simulink model "Distribuition"  (R2024a)
settings: Solver=VariableStepAuto  StartTime=0.0  StopTime=10.0  RelTol=1e-3
InitFcn:
  | % Exemplo no Windows, usando pscp (PuTTY scp) ou scp no Linux/macOS
  | chave = 'C:/Users/guilh/OneDrive/Área de Trabalho/matlab-Gemeo/Sombra_Distribution/Matlab_conect/id_rsa_matlab';
  | usuario = 'root';
  | ip = '200.145.26.206';
  | arquivo_remoto = '/root/ProjetoGemeo/AAS/Distribution/Variables.csv';
  | arquivo_local = 'Variables.csv';
  | 
  | % Comando scp para baixar arquivo usando chave privada
  | cmd = sprintf('scp -i "%s" %s@%s:"%s" "%s"', chave, usuario, ip, arquivo_remoto);
  | 
  | % Executar comando no sistema
  | [status, cmdout] = system(cmd);
  | 
  | if status == 0
  |     disp('Download concluído via SCP externo!');
  | else
  |     disp('Erro ao executar SCP:');
  |     disp(cmdout);
  | end
  | 
  | tabela = readtable('Variables.csv', 'Delimiter', ';');
  | nomesVariaveis = tabela.Variable;
libraries: opclib x1, opcualib x1
settings Model: Creator=guilh  LastModifiedBy=guilh

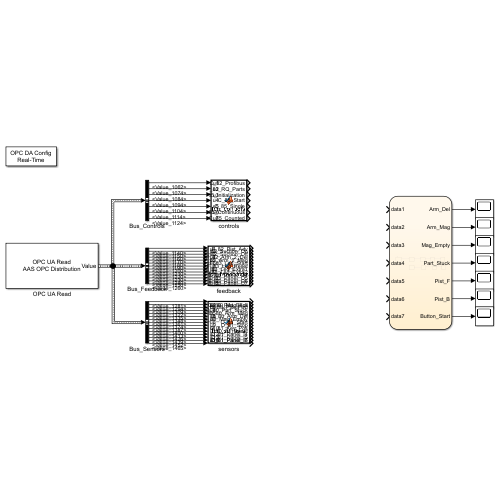
[thumbnail: Simulink's stored preview of the top-level diagram]
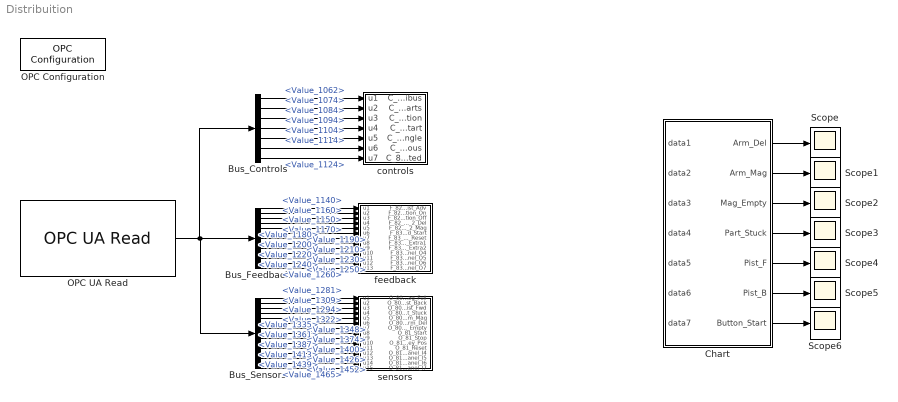
== system Distribuition ==
  Bus_Controls : BusSelector  OutputSignals=Value_1062,Value_1074,Value_1084,Value_1094,Value_1104,Value_1114,Value_1124
  Bus_Feedback : BusSelector  OutputSignals=Value_1140,Value_1150,Value_1160,Value_1170,Value_1180,Value_1190,Value_1200,Value_1210,Value_1220,Value_1230,Value_1240,Value_1250,Value_1260
  Bus_Sensors : BusSelector  OutputSignals=Value_1281,Value_1294,Value_1309,Value_1322,Value_1335,Value_1348,Value_1361,Value_1374,Value_1387,Value_1400,Value_1413,Value_1426,Value_1439,Value_1452,Value_1465
  Chart : Stateflow chart  TreatAsAtomicUnit=on
  OPC Configuration : opclib/OPC Configuration  errMissingItems=Error  errReadWrite=Warn  errShutdown=Error  errRTViolation=Warn  rtEnable=on  speedup=1  showLatency=off  beingUsed=on
  OPC UA Read : opcualib/OPC UA Read  SelectedServer=AAS OPC Distribution  ServerList=AAS OPC Distribution  NodeList={ '1', 'Value', '6', '1062', '1'; '2', 'Value', '6', '1074', '1'; '3', 'Value', '6', '1084', '1'; '4', 'Value', '6', '1094', '1'; '5', 'Value', '6', '1104', '1'; '6', 'Value', '6', '1114', '1'; '7', 'Value', '6', '1124', '1'; '8', 'Value', '6', '1140', '1'; '9', 'Value', '6', '1150', '1'; '10', 'Value', '6', '1160', '1'; '11', 'Value', '6', '1170', '1'; '12', 'Value', '6', '1180', '1'; '13', 'Value', '6', '1190', '1'; '14', 'Value', '6', '1200', '1'; '15', 'Value', '6', '1210', '1'; '16', 'Value', '6', '1220', '1'; '17', 'Value', '6', '1230', '1'; '18', 'Value', '6', '1240', '1'; '19', 'Value', '6', '1250', '1'; '20', 'Value', '6', '1260', '1'; '21', 'Value', '6', '1281', '1'; '22', 'Value', '6', '1294', '1'; '23', 'Value', '6', '1309', '1'; '24', 'Value', '6', '1322', '1'; '25', 'Value', '6', '1335', '1'; '26', 'Value', '6', '1348', '1'; '27', 'Value', '6', '1361', '1'; '28', 'Value', '6', '1374', '1'; '29', 'Value', '6', '1387', '1'; '30', 'Value', '6', '1400', '1'; '31', 'Value', '6', '1413', '1'; '32', 'Value', '6', '1426', '1'; '33', 'Value', '6', '1439', '1'; '34', 'Value', '6', '1452', '1'; '35', 'Value', '6', '1465', '1' }  ShowQualityPort=off  ShowTimestampPort=off  ShowTimestampPortAs=Seconds since start  SampleTime=-1
  Scope{,1..6} (7 alike) : Scope
  controls : MATLAB Function  TreatAsAtomicUnit=on
  feedback : MATLAB Function  TreatAsAtomicUnit=on
  sensors : MATLAB Function  TreatAsAtomicUnit=on
  wires:
  Chart/1(Arm_Del) -> Scope/1
  Chart/2(Arm_Mag) -> Scope1/1
  Chart/3(Mag_Empty) -> Scope2/1
  Chart/4(Part_Stuck) -> Scope3/1
  Chart/5(Pist_F) -> Scope4/1
  Chart/6(Pist_B) -> Scope5/1
  Chart/7(Button_Start) -> Scope6/1
  OPC UA Read/1 -> Bus_Sensors/1, Bus_Feedback/1, Bus_Controls/1
  Bus_Controls/7 -> controls/7(u7)  "<Value_1124>"
  Bus_Controls/6 -> controls/6(u6)  "<Value_1114>"
  Bus_Controls/5 -> controls/5(u5)  "<Value_1104>"
  Bus_Controls/4 -> controls/4(u4)  "<Value_1094>"
  Bus_Controls/3 -> controls/3(u3)  "<Value_1084>"
  Bus_Controls/2 -> controls/2(u2)  "<Value_1074>"
  Bus_Controls/1 -> controls/1(u1)  "<Value_1062>"
  Bus_Feedback/1 -> feedback/1(u1)  "<Value_1140>"
  Bus_Feedback/2 -> feedback/2(u2)  "<Value_1150>"
  Bus_Feedback/3 -> feedback/3(u3)  "<Value_1160>"
  Bus_Feedback/4 -> feedback/4(u4)  "<Value_1170>"
  Bus_Feedback/5 -> feedback/5(u5)  "<Value_1180>"
  Bus_Feedback/6 -> feedback/6(u6)  "<Value_1190>"
  Bus_Feedback/7 -> feedback/7(u7)  "<Value_1200>"
  Bus_Feedback/8 -> feedback/8(u8)  "<Value_1210>"
  Bus_Feedback/9 -> feedback/9(u9)  "<Value_1220>"
  Bus_Feedback/10 -> feedback/10(u10)  "<Value_1230>"
  Bus_Feedback/11 -> feedback/11(u11)  "<Value_1240>"
  Bus_Feedback/12 -> feedback/12(u12)  "<Value_1250>"
  Bus_Feedback/13 -> feedback/13(u13)  "<Value_1260>"
  Bus_Sensors/1 -> sensors/1(u1)  "<Value_1281>"
  Bus_Sensors/2 -> sensors/2(u2)  "<Value_1294>"
  Bus_Sensors/3 -> sensors/3(u3)  "<Value_1309>"
  Bus_Sensors/4 -> sensors/4(u4)  "<Value_1322>"
  Bus_Sensors/5 -> sensors/5(u5)  "<Value_1335>"
  Bus_Sensors/6 -> sensors/6(u6)  "<Value_1348>"
  Bus_Sensors/7 -> sensors/7(u7)  "<Value_1361>"
  Bus_Sensors/8 -> sensors/8(u8)  "<Value_1374>"
  Bus_Sensors/9 -> sensors/9(u9)  "<Value_1387>"
  Bus_Sensors/10 -> sensors/10(u10)  "<Value_1400>"
  Bus_Sensors/11 -> sensors/11(u11)  "<Value_1413>"
  Bus_Sensors/12 -> sensors/12(u12)  "<Value_1426>"
  Bus_Sensors/13 -> sensors/13(u13)  "<Value_1439>"
  Bus_Sensors/14 -> sensors/14(u14)  "<Value_1452>"
  Bus_Sensors/15 -> sensors/15(u15)  "<Value_1465>"

== matlab function Distribuition/sensors ==
  data: u1 input; u2 input; u3 input; u4 input; u5 input; u6 input; u7 input; u8 input; u9 input; u10 input; u11 input; u12 input; u13 input; u14 input; u15 input; O_80_Mag_Full output; O_80_Pist_Back output; O_80_Pist_Fwd output; O_80_Part_Stuck output; O_80_Arm_Mag output; O_80_Arm_Del output; O_80_Mag_Empty output; O_81_Start output; O_81_Stop output; O_81_Key_Pos output; O_81_Reset output; O_81_Panel_I4 output; O_81_Panel_I5 output; O_81_Panel_I6 output; O_81_Panel_I7 output
function [O_80_Mag_Full,O_80_Pist_Back,O_80_Pist_Fwd,O_80_Part_Stuck,...
    O_80_Arm_Mag,O_80_Arm_Del,O_80_Mag_Empty,O_81_Start,O_81_Stop,...
    O_81_Key_Pos,O_81_Reset,O_81_Panel_I4,O_81_Panel_I5,O_81_Panel_I6,...
    O_81_Panel_I7] = fcn_sensors(u1,u2,u3,u4,u5,u6,u7,u8,u9,...
    u10,u11,u12,u13,u14,u15)

O_80_Mag_Full = u1;
O_80_Pist_Back = u2;
O_80_Pist_Fwd = u3;
O_80_Part_Stuck = u4;
O_80_Arm_Mag = u5;
O_80_Arm_Del = u6;
O_80_Mag_Empty = u7;
O_81_Start = u8;
O_81_Stop = u9;
O_81_Key_Pos = u10;
O_81_Reset = u11;
O_81_Panel_I4 = u12;
O_81_Panel_I5 = u13;
O_81_Panel_I6 = u14;
O_81_Panel_I7 = u15;

== matlab function Distribuition/feedback ==
  data: u1 input; F_82_Pist_Adv output; u2 input; u3 input; u4 input; u5 input; u6 input; u7 input; u8 input; u9 input; u10 input; u11 input; u12 input; u13 input; F_82_Suction_On output; F_82_Suction_Off output; F_82_Arm_2_Del output; F_82_Arm_2_Mag output; F_83_Led_Start output; F_83_Led_Reset output; F_83_Led_Extra1 output; F_83_Led_Extra2 output; F_83_Panel_O4 output; F_83_Panel_O5 output; F_83_Panel_O6 output; F_83_Panel_O7 output
function [F_82_Pist_Adv,F_82_Suction_On,F_82_Suction_Off,F_82_Arm_2_Del, ...
    F_82_Arm_2_Mag,F_83_Led_Start,F_83_Led_Reset,F_83_Led_Extra1,...
    F_83_Led_Extra2,F_83_Panel_O4,F_83_Panel_O5,F_83_Panel_O6,...
    F_83_Panel_O7] = fcn_feedbacks(u1,u2,u3,u4,u5,u6,u7,u8,u9,...
    u10,u11,u12,u13)

F_82_Pist_Adv = u1;
F_82_Suction_On = u2;
F_82_Suction_Off = u3;
F_82_Arm_2_Del = u4;
F_82_Arm_2_Mag = u5;
F_83_Led_Start = u6;
F_83_Led_Reset = u7;
F_83_Led_Extra1 = u8;
F_83_Led_Extra2 = u9;
F_83_Panel_O4 = u10;
F_83_Panel_O5 = u11;
F_83_Panel_O6 = u12;
F_83_Panel_O7 = u13;

== matlab function Distribuition/controls ==
  data: u1 input; u2 input; u3 input; u4 input; u5 input; u6 input; u7 input; C_82_Profibus output; C_83_RQ_Parts output; C_85_Initialization output; C_85_Start output; C_85_Single output; C_85_Continuous output; C_85_Counted output
function [C_82_Profibus, C_83_RQ_Parts, ...
    C_85_Initialization, C_85_Start, ...
    C_85_Single, C_85_Continuous, ...
    C_85_Counted] = fcn_controls(u1,u2,u3,u4,u5,u6,u7)

C_82_Profibus = u1;
C_83_RQ_Parts = u2;
C_85_Initialization = u3;
C_85_Start = u4;
C_85_Single = u5; 
C_85_Continuous = u6;
C_85_Counted = u7;

== stateflow chart Distribuition/Chart ==
  state Init
    entry:
    Button_Start = data7;
    Pist_B = data1;
    Pist_F = data2;
    Part_Stuck = data3;
    Arm_Mag = data4;
    Arm_Del = data5;
    Mag_Empty = data6;
  state Arm_2_Del
    entry:
    Pist_B = 1;
    Pist_F = 0;
    Part_Stuck = 0;
    Arm_Mag = 0;
    Arm_Del = 1;
    Mag_Empty = 0;
  state Pist_Fowd
    entry:
    Pist_B = 0;
    Pist_F = 1;
    Part_Stuck = 0;
    Arm_Mag = 0;
    Arm_Del = 1;
    Mag_Empty = 0;
  state Pist_Back
    entry:
    Pist_B = 1;
    Pist_F = 0;
    Part_Stuck = 0;
    Arm_Mag = 0;
    Arm_Del = 1;
    Mag_Empty = 0;
  state Arm_2_Mag
    entry:
    Pist_B = 1;
    Pist_F = 0;
    Part_Stuck = 0;
    Arm_Mag = 1;
    Arm_Del = 0;
    Mag_Empty = 0;
  state Arm_2_Mag1
    entry:
    Button_Start = 0;
    Pist_B = 1;
    Pist_F = 0;
    Part_Stuck = 0;
    Arm_Mag = 1;
    Arm_Del = 0;
    Mag_Empty = 0;
  state Stuck_Off
    entry:
    Pist_B = 1;
    Pist_F = 0;
    Part_Stuck = 0;
    Arm_Mag = 0;
    Arm_Del = 1;
    Mag_Empty = 0;
  state Arm_2_Del1
    entry:
    Pist_B = 1;
    Pist_F = 0;
    Part_Stuck = 1;
    Arm_Mag = 0;
    Arm_Del = 1;
    Mag_Empty = 0;
  state Stuck_On
    entry:
    Pist_B = 1;
    Pist_F = 0;
    Part_Stuck = 1;
    Arm_Mag = 1;
    Arm_Del = 0;
    Mag_Empty = 0;
  (default) -> Init
  Arm_2_Del -> Pist_Fowd : [Arm_Mag == 0 && Arm_Del == 1]
  Pist_Fowd -> Pist_Back : [Pist_B == 0 && Pist_F == 1]
  Pist_Back -> Arm_2_Mag : [Pist_B == 1 && Pist_F == 0]
  Init -> Arm_2_Del : [Button_Start == 1 && Mag_Empty == 0]
  Arm_2_Mag -> Stuck_On : [Arm_Mag == 1 && Arm_Del == 0]
  Arm_2_Del1 -> Stuck_Off : [Arm_Mag == 0 && Arm_Del == 1]
  Stuck_On -> Arm_2_Del1 : [Part_Stuck == 1]
  Stuck_Off -> Arm_2_Mag1 : [Part_Stuck == 0]
  data: data1 input; data2 input; data3 input; data4 input; data5 input; data6 input; Arm_Del output; Arm_Mag output; Mag_Empty output; Part_Stuck output; Pist_F output; Pist_B output; data7 input; Button_Start output
